simulink model "PassStRclCmdSrvCal"  (R2024b)
settings: Solver=FixedStepDiscrete  StartTime=0.0  StopTime=10.0  FixedStep=0.01  RelTol=1e-3
undefined symbols (not defined in the file or in its folder): KeSMSwPosInvalidVal_Val, PowerMode1
settings Model: ModifiedHistory=2024.7.9 V3.0.0 557模式流程V1.9  Creator=sn2xws  LastModifiedBy=sn55gm
settings SolverCC: AlgebraicLoopSolver=TrustRegion
settings DataIOCC: SaveFormat=StructureWithTime  ReturnWorkspaceOutputs=off
settings OptimizationCC: DefaultParameterBehavior=Inlined  EnhancedBackFolding=on  PassReuseOutputArgsAs=Individual arguments  ZeroExternalMemoryAtStartup=off  ZeroInternalMemoryAtStartup=off  OptimizeBlockOrder=speed  DifferentSizesBufferReuse=on  OptimizationCustomize=off  EfficientTunableParamExpr=on
settings DebuggingCC: ParameterTunabilityLossMsg=error  UnconnectedInputMsg=warning  UnconnectedOutputMsg=warning  UnconnectedLineMsg=warning  ArithmeticOperatorsInVariantConditions=warning
settings ModelReferenceCC: EnableRefExpFcnMdlSchedulingChecks=on  ModelReferenceNumInstancesAllowed=Single
settings SFSimCC: MATLABDynamicMemAlloc=off  CustomCodeUndefinedFunction=UseInterfaceOnly
settings RTWCC: Description=AUTOSAR  SystemTargetFile=autosar.tlc  GenCodeOnly=on  TemplateMakefile=ert_default_tmf  GenerateReport=on  IncludeHyperlinkInReport=on  LaunchReport=on  DataTypeReplacement=CDataTypesFixedWidth  GenerateTraceInfo=on  GenerateTraceReport=on  GenerateTraceReportSl=on  GenerateTraceReportSf=on  GenerateTraceReportEml=on  GenerateCodeMetricsReport=on  GPUComputeCapability=3.5
settings CodeAppCC: ForceParamTrailComments=on  IgnoreCustomStorageClasses=off  OperatorAnnotations=on  SimulinkDataObjDesc=on  SFDataObjDesc=on  InsertBlockDesc=on
settings STFCustomTargetCC: TargetLangStandard=C99 (ISO)  MultiwordLength=256  ParMdlRefBuildCompliant=on  CompOptLevelCompliant=on  IncludeMdlTerminateFcn=off  CombineOutputUpdateFcns=on  SuppressErrorStatus=on  ERTCustomFileBanners=on  SupportNonFinite=off  SupportComplex=off  SupportContinuousTime=off  SupportNonInlinedSFcns=off  RemoveResetFunc=on  MATLABClassNameForMDSCustomization=Simulink.SoftwareTarget.ERTCustomization  AutosarCompliant=on  UseToolchainInfoCompliant=on  LookupTableObjectStructAxisOrder=2,1,3,4,...  LUTObjectStructOrderEvenSpacing=Size,Table,Breakpoints  SystemTargetFile=autosar.tlc
settings ERTTargetCC: TargetLangStandard=C99 (ISO)  ConcurrentExecutionCompliant=off  IncludeMdlTerminateFcn=off  SuppressErrorStatus=on  SupportNonFinite=off  SupportComplex=off  ModelStepFunctionPrototypeControlCompliant=off  CPPClassGenCompliant=off  AutosarCompliant=on  LookupTableObjectStructAxisOrder=2,1,3,4,...  LUTObjectStructOrderEvenSpacing=Size,Table,Breakpoints  ERTCustomFileTemplate=example_file_process.tlc  ERTFilePackagingFormat=Compact  BooleanTrueId=TRUE  BooleanFalseId=FALSE  DynamicArrayContainerType=coder::array

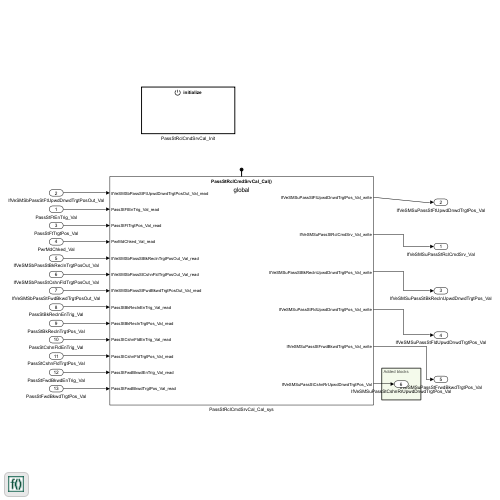
[thumbnail: Simulink's stored preview of the top-level diagram]
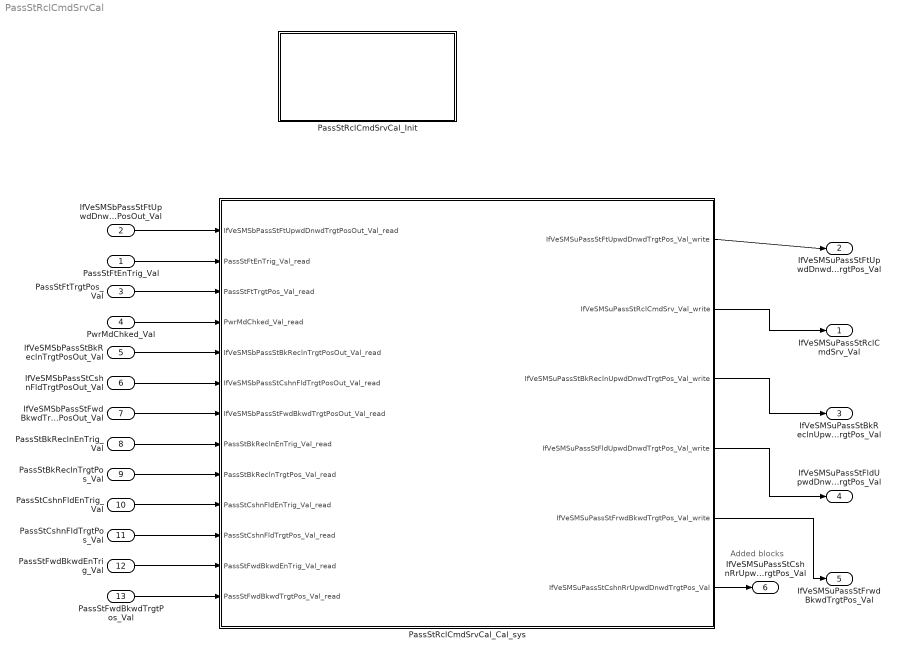
== system PassStRclCmdSrvCal ==
  note: Added blocks
  PassStFtEnTrig_Val : Inport  OutDataTypeStr=boolean  PortDimensions=1
  IfVeSMSbPassStFtUpwdDnwdTrgtPosOut_Val : Inport  Port=2  OutDataTypeStr=boolean  PortDimensions=1
  PassStFtTrgtPos_Val : Inport  Port=3  OutDataTypeStr=uint16  PortDimensions=1
  PwrMdChked_Val : Inport  Port=4  OutDataTypeStr=Enum: PowerMode1  PortDimensions=1
  IfVeSMSbPassStBkReclnTrgtPosOut_Val : Inport  Port=5  OutDataTypeStr=boolean  PortDimensions=1
  IfVeSMSbPassStCshnFldTrgtPosOut_Val : Inport  Port=6  OutDataTypeStr=boolean  PortDimensions=1
  IfVeSMSbPassStFwdBkwdTrgtPosOut_Val : Inport  Port=7  OutDataTypeStr=boolean  PortDimensions=1
  PassStBkReclnEnTrig_Val : Inport  Port=8  OutDataTypeStr=boolean  PortDimensions=1
  PassStBkReclnTrgtPos_Val : Inport  Port=9  OutDataTypeStr=uint16  PortDimensions=1
  PassStCshnFldEnTrig_Val : Inport  Port=10  OutDataTypeStr=boolean  PortDimensions=1
  PassStCshnFldTrgtPos_Val : Inport  Port=11  OutDataTypeStr=uint16  PortDimensions=1
  PassStFwdBkwdEnTrig_Val : Inport  Port=12  OutDataTypeStr=boolean  PortDimensions=1
  PassStFwdBkwdTrgtPos_Val : Inport  Port=13  OutDataTypeStr=uint16  PortDimensions=1
  PassStRclCmdSrvCal_Cal_sys : Subsystem
  PassStRclCmdSrvCal_Init : Subsystem
  IfVeSMSuPassStRclCmdSrv_Val : Outport  OutDataTypeStr=boolean  PortDimensions=1  VectorParamsAs1DForOutWhenUnconnected=off
  IfVeSMSuPassStFtUpwdDnwdTrgtPos_Val : Outport  Port=2  OutDataTypeStr=uint16  PortDimensions=1  VectorParamsAs1DForOutWhenUnconnected=off
  IfVeSMSuPassStBkReclnUpwdDnwdTrgtPos_Val : Outport  Port=3  OutDataTypeStr=uint16  PortDimensions=1  VectorParamsAs1DForOutWhenUnconnected=off
  IfVeSMSuPassStFldUpwdDnwdTrgtPos_Val : Outport  Port=4  OutDataTypeStr=uint16  PortDimensions=1  VectorParamsAs1DForOutWhenUnconnected=off
  IfVeSMSuPassStFrwdBkwdTrgtPos_Val : Outport  Port=5  OutDataTypeStr=uint16  PortDimensions=1  VectorParamsAs1DForOutWhenUnconnected=off
  IfVeSMSuPassStCshnRrUpwdDnwdTrgtPos_Val : Outport  Port=6  OutDataTypeStr=uint16  PortDimensions=1
  wires:
  PassStRclCmdSrvCal_Cal_sys/1(IfVeSMSuPassStFtUpwdDnwdTrgtPos_Val_write) -> IfVeSMSuPassStFtUpwdDnwdTrgtPos_Val/1
  PassStRclCmdSrvCal_Cal_sys/2(IfVeSMSuPassStRclCmdSrv_Val_write) -> IfVeSMSuPassStRclCmdSrv_Val/1
  PassStFtTrgtPos_Val/1 -> PassStRclCmdSrvCal_Cal_sys/3(PassStFtTrgtPos_Val_read)
  IfVeSMSbPassStFtUpwdDnwdTrgtPosOut_Val/1 -> PassStRclCmdSrvCal_Cal_sys/1(IfVeSMSbPassStFtUpwdDnwdTrgtPosOut_Val_read)
  PassStFtEnTrig_Val/1 -> PassStRclCmdSrvCal_Cal_sys/2(PassStFtEnTrig_Val_read)
  PwrMdChked_Val/1 -> PassStRclCmdSrvCal_Cal_sys/4(PwrMdChked_Val_read)
  IfVeSMSbPassStBkReclnTrgtPosOut_Val/1 -> PassStRclCmdSrvCal_Cal_sys/5(IfVeSMSbPassStBkReclnTrgtPosOut_Val_read)
  IfVeSMSbPassStCshnFldTrgtPosOut_Val/1 -> PassStRclCmdSrvCal_Cal_sys/6(IfVeSMSbPassStCshnFldTrgtPosOut_Val_read)
  IfVeSMSbPassStFwdBkwdTrgtPosOut_Val/1 -> PassStRclCmdSrvCal_Cal_sys/7(IfVeSMSbPassStFwdBkwdTrgtPosOut_Val_read)
  PassStBkReclnEnTrig_Val/1 -> PassStRclCmdSrvCal_Cal_sys/8(PassStBkReclnEnTrig_Val_read)
  PassStBkReclnTrgtPos_Val/1 -> PassStRclCmdSrvCal_Cal_sys/9(PassStBkReclnTrgtPos_Val_read)
  PassStCshnFldEnTrig_Val/1 -> PassStRclCmdSrvCal_Cal_sys/10(PassStCshnFldEnTrig_Val_read)
  PassStCshnFldTrgtPos_Val/1 -> PassStRclCmdSrvCal_Cal_sys/11(PassStCshnFldTrgtPos_Val_read)
  PassStFwdBkwdEnTrig_Val/1 -> PassStRclCmdSrvCal_Cal_sys/12(PassStFwdBkwdEnTrig_Val_read)
  PassStFwdBkwdTrgtPos_Val/1 -> PassStRclCmdSrvCal_Cal_sys/13(PassStFwdBkwdTrgtPos_Val_read)
  PassStRclCmdSrvCal_Cal_sys/3(IfVeSMSuPassStBkReclnUpwdDnwdTrgtPos_Val_write) -> IfVeSMSuPassStBkReclnUpwdDnwdTrgtPos_Val/1
  PassStRclCmdSrvCal_Cal_sys/4(IfVeSMSuPassStFldUpwdDnwdTrgtPos_Val_write) -> IfVeSMSuPassStFldUpwdDnwdTrgtPos_Val/1
  PassStRclCmdSrvCal_Cal_sys/5(IfVeSMSuPassStFrwdBkwdTrgtPos_Val_write) -> IfVeSMSuPassStFrwdBkwdTrgtPos_Val/1
  PassStRclCmdSrvCal_Cal_sys/6(IfVeSMSuPassStCshnRrUpwdDnwdTrgtPos_Val) -> IfVeSMSuPassStCshnRrUpwdDnwdTrgtPos_Val/1

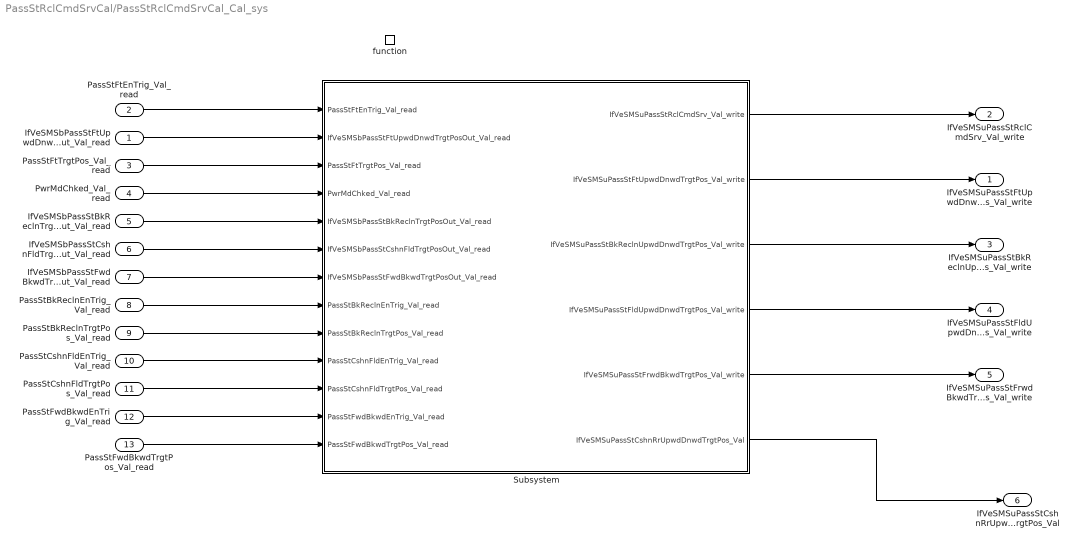
== system PassStRclCmdSrvCal/PassStRclCmdSrvCal_Cal_sys ==
  IfVeSMSbPassStFtUpwdDnwdTrgtPosOut_Val_read : Inport
  PassStFtEnTrig_Val_read : Inport  Port=2
  PassStFtTrgtPos_Val_read : Inport  Port=3
  PwrMdChked_Val_read : Inport  Port=4
  IfVeSMSbPassStBkReclnTrgtPosOut_Val_read : Inport  Port=5
  IfVeSMSbPassStCshnFldTrgtPosOut_Val_read : Inport  Port=6
  IfVeSMSbPassStFwdBkwdTrgtPosOut_Val_read : Inport  Port=7
  PassStBkReclnEnTrig_Val_read : Inport  Port=8
  PassStBkReclnTrgtPos_Val_read : Inport  Port=9
  PassStCshnFldEnTrig_Val_read : Inport  Port=10
  PassStCshnFldTrgtPos_Val_read : Inport  Port=11
  PassStFwdBkwdEnTrig_Val_read : Inport  Port=12
  PassStFwdBkwdTrgtPos_Val_read : Inport  Port=13
  function : TriggerPort  TriggerType=function-call  IsSimulinkFunction=on  FunctionName=PassStRclCmdSrvCal_Cal  VariantControl=(inherit)
  Subsystem : Subsystem
  IfVeSMSuPassStFtUpwdDnwdTrgtPos_Val_write : Outport  VectorParamsAs1DForOutWhenUnconnected=off
      settings: EnsureOutportIsVirtual=on
  IfVeSMSuPassStRclCmdSrv_Val_write : Outport  Port=2  VectorParamsAs1DForOutWhenUnconnected=off
      settings: EnsureOutportIsVirtual=on
  IfVeSMSuPassStBkReclnUpwdDnwdTrgtPos_Val_write : Outport  Port=3  VectorParamsAs1DForOutWhenUnconnected=off
      settings: EnsureOutportIsVirtual=on
  IfVeSMSuPassStFldUpwdDnwdTrgtPos_Val_write : Outport  Port=4  VectorParamsAs1DForOutWhenUnconnected=off
      settings: EnsureOutportIsVirtual=on
  IfVeSMSuPassStFrwdBkwdTrgtPos_Val_write : Outport  Port=5  VectorParamsAs1DForOutWhenUnconnected=off
      settings: EnsureOutportIsVirtual=on
  IfVeSMSuPassStCshnRrUpwdDnwdTrgtPos_Val : Outport  Port=6
      settings: EnsureOutportIsVirtual=on
  wires:
  Subsystem/1(IfVeSMSuPassStRclCmdSrv_Val_write) -> IfVeSMSuPassStRclCmdSrv_Val_write/1
  Subsystem/2(IfVeSMSuPassStFtUpwdDnwdTrgtPos_Val_write) -> IfVeSMSuPassStFtUpwdDnwdTrgtPos_Val_write/1
  PassStFtEnTrig_Val_read/1 -> Subsystem/1(PassStFtEnTrig_Val_read)
  IfVeSMSbPassStFtUpwdDnwdTrgtPosOut_Val_read/1 -> Subsystem/2(IfVeSMSbPassStFtUpwdDnwdTrgtPosOut_Val_read)
  PassStFtTrgtPos_Val_read/1 -> Subsystem/3(PassStFtTrgtPos_Val_read)
  PwrMdChked_Val_read/1 -> Subsystem/4(PwrMdChked_Val_read)
  IfVeSMSbPassStBkReclnTrgtPosOut_Val_read/1 -> Subsystem/5(IfVeSMSbPassStBkReclnTrgtPosOut_Val_read)
  IfVeSMSbPassStCshnFldTrgtPosOut_Val_read/1 -> Subsystem/6(IfVeSMSbPassStCshnFldTrgtPosOut_Val_read)
  IfVeSMSbPassStFwdBkwdTrgtPosOut_Val_read/1 -> Subsystem/7(IfVeSMSbPassStFwdBkwdTrgtPosOut_Val_read)
  PassStBkReclnEnTrig_Val_read/1 -> Subsystem/8(PassStBkReclnEnTrig_Val_read)
  PassStBkReclnTrgtPos_Val_read/1 -> Subsystem/9(PassStBkReclnTrgtPos_Val_read)
  PassStCshnFldEnTrig_Val_read/1 -> Subsystem/10(PassStCshnFldEnTrig_Val_read)
  PassStCshnFldTrgtPos_Val_read/1 -> Subsystem/11(PassStCshnFldTrgtPos_Val_read)
  PassStFwdBkwdEnTrig_Val_read/1 -> Subsystem/12(PassStFwdBkwdEnTrig_Val_read)
  PassStFwdBkwdTrgtPos_Val_read/1 -> Subsystem/13(PassStFwdBkwdTrgtPos_Val_read)
  Subsystem/3(IfVeSMSuPassStBkReclnUpwdDnwdTrgtPos_Val_write) -> IfVeSMSuPassStBkReclnUpwdDnwdTrgtPos_Val_write/1
  Subsystem/4(IfVeSMSuPassStFldUpwdDnwdTrgtPos_Val_write) -> IfVeSMSuPassStFldUpwdDnwdTrgtPos_Val_write/1
  Subsystem/5(IfVeSMSuPassStFrwdBkwdTrgtPos_Val_write) -> IfVeSMSuPassStFrwdBkwdTrgtPos_Val_write/1
  Subsystem/6(IfVeSMSuPassStCshnRrUpwdDnwdTrgtPos_Val) -> IfVeSMSuPassStCshnRrUpwdDnwdTrgtPos_Val/1

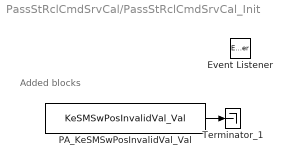
== system PassStRclCmdSrvCal/PassStRclCmdSrvCal_Init ==
  note: Added blocks
  Event Listener : EventListener  EventName=reset
  PA_KeSMSwPosInvalidVal_Val : Constant  Value=KeSMSwPosInvalidVal_Val
  Terminator_1 : Terminator
  wires:
  PA_KeSMSwPosInvalidVal_Val/1 -> Terminator_1/1

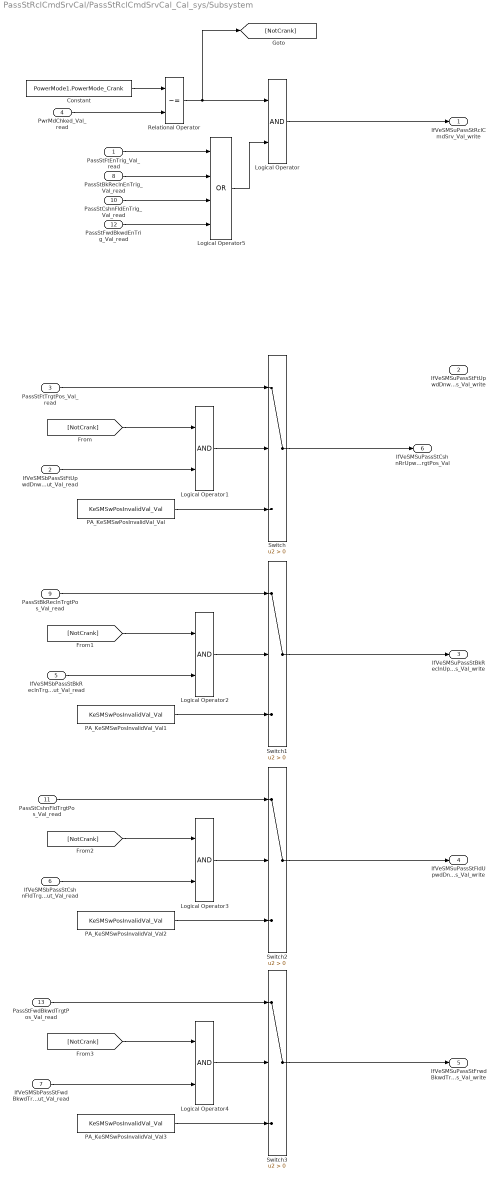
== system PassStRclCmdSrvCal/PassStRclCmdSrvCal_Cal_sys/Subsystem ==
  PassStFtEnTrig_Val_read : Inport
  IfVeSMSbPassStFtUpwdDnwdTrgtPosOut_Val_read : Inport  Port=2
  PassStFtTrgtPos_Val_read : Inport  Port=3
  PwrMdChked_Val_read : Inport  Port=4
  IfVeSMSbPassStBkReclnTrgtPosOut_Val_read : Inport  Port=5
  IfVeSMSbPassStCshnFldTrgtPosOut_Val_read : Inport  Port=6
  IfVeSMSbPassStFwdBkwdTrgtPosOut_Val_read : Inport  Port=7
  PassStBkReclnEnTrig_Val_read : Inport  Port=8
  PassStBkReclnTrgtPos_Val_read : Inport  Port=9
  PassStCshnFldEnTrig_Val_read : Inport  Port=10
  PassStCshnFldTrgtPos_Val_read : Inport  Port=11
  PassStFwdBkwdEnTrig_Val_read : Inport  Port=12
  PassStFwdBkwdTrgtPos_Val_read : Inport  Port=13
  Constant : Constant  Value=PowerMode1.PowerMode_Crank  OutDataTypeStr=Enum: PowerMode1
  Logical Operator{,1..4} (5 alike) : Logic  AllPortsSameDT=off  OutDataTypeStr=boolean
  Logical Operator5 : Logic  Operator=OR  Inputs=4  AllPortsSameDT=off  OutDataTypeStr=boolean
  PA_KeSMSwPosInvalidVal_Val{,1..3} (4 alike) : Constant  Value=KeSMSwPosInvalidVal_Val
  Relational Operator : RelationalOperator  Operator=~=  OutDataTypeStr=boolean  RndMeth=Simplest  InputSameDT=off
  Switch{,1..3} (4 alike) : Switch  Criteria=u2 > Threshold  SaturateOnIntegerOverflow=off  InputSameDT=off
  IfVeSMSuPassStRclCmdSrv_Val_write : Outport  VectorParamsAs1DForOutWhenUnconnected=off
      settings: EnsureOutportIsVirtual=on
  IfVeSMSuPassStFtUpwdDnwdTrgtPos_Val_write : Outport  Port=2  VectorParamsAs1DForOutWhenUnconnected=off
      settings: EnsureOutportIsVirtual=on
  IfVeSMSuPassStBkReclnUpwdDnwdTrgtPos_Val_write : Outport  Port=3  VectorParamsAs1DForOutWhenUnconnected=off
      settings: EnsureOutportIsVirtual=on
  IfVeSMSuPassStFldUpwdDnwdTrgtPos_Val_write : Outport  Port=4  VectorParamsAs1DForOutWhenUnconnected=off
      settings: EnsureOutportIsVirtual=on
  IfVeSMSuPassStFrwdBkwdTrgtPos_Val_write : Outport  Port=5  VectorParamsAs1DForOutWhenUnconnected=off
      settings: EnsureOutportIsVirtual=on
  IfVeSMSuPassStCshnRrUpwdDnwdTrgtPos_Val : Outport  Port=6
  wires:
  PA_KeSMSwPosInvalidVal_Val/1 -> Switch/3
  PassStFtTrgtPos_Val_read/1 -> Switch/1
  PwrMdChked_Val_read/1 -> Relational Operator/2
  Constant/1 -> Relational Operator/1
  Logical Operator/1 -> IfVeSMSuPassStRclCmdSrv_Val_write/1
  Relational Operator/1 -> [NotCrank], Logical Operator/1
  Logical Operator1/1 -> Switch/2
  IfVeSMSbPassStFtUpwdDnwdTrgtPosOut_Val_read/1 -> Logical Operator1/2
  [NotCrank] -> Logical Operator1/1
  Switch3/1 -> IfVeSMSuPassStFrwdBkwdTrgtPos_Val_write/1
  Switch2/1 -> IfVeSMSuPassStFldUpwdDnwdTrgtPos_Val_write/1
  Switch1/1 -> IfVeSMSuPassStBkReclnUpwdDnwdTrgtPos_Val_write/1
  [NotCrank] -> Logical Operator2/1
  Logical Operator2/1 -> Switch1/2
  PA_KeSMSwPosInvalidVal_Val1/1 -> Switch1/3
  Logical Operator3/1 -> Switch2/2
  PA_KeSMSwPosInvalidVal_Val2/1 -> Switch2/3
  [NotCrank] -> Logical Operator3/1
  Logical Operator4/1 -> Switch3/2
  PA_KeSMSwPosInvalidVal_Val3/1 -> Switch3/3
  [NotCrank] -> Logical Operator4/1
  IfVeSMSbPassStBkReclnTrgtPosOut_Val_read/1 -> Logical Operator2/2
  PassStBkReclnTrgtPos_Val_read/1 -> Switch1/1
  IfVeSMSbPassStCshnFldTrgtPosOut_Val_read/1 -> Logical Operator3/2
  PassStCshnFldTrgtPos_Val_read/1 -> Switch2/1
  IfVeSMSbPassStFwdBkwdTrgtPosOut_Val_read/1 -> Logical Operator4/2
  PassStFwdBkwdTrgtPos_Val_read/1 -> Switch3/1
  Logical Operator5/1 -> Logical Operator/2
  PassStFtEnTrig_Val_read/1 -> Logical Operator5/1
  PassStBkReclnEnTrig_Val_read/1 -> Logical Operator5/2
  PassStCshnFldEnTrig_Val_read/1 -> Logical Operator5/3
  PassStFwdBkwdEnTrig_Val_read/1 -> Logical Operator5/4
  Switch/1 -> IfVeSMSuPassStCshnRrUpwdDnwdTrgtPos_Val/1
